simulink model "hardware1"  (R2018a)
settings: Solver=VariableStepAuto  StartTime=0.0  StopTime=10000  RelTol=1e-3
model workspace (MAT data in the model file):
  D = Simulink.Parameter
  D.DataType = 'auto'
  D.Dimensions = [0 0]
libraries: powerlib x15, simulink x1, powerlib_meascontrol x1
settings Model: Creator=yusuf  LastModifiedBy=yusuf

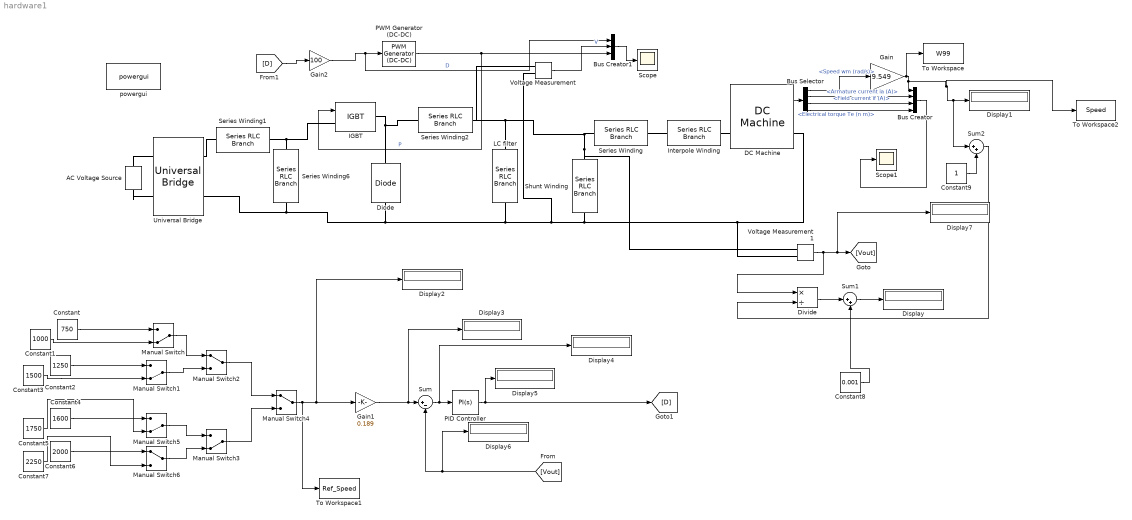
== system hardware1 ==
  AC Voltage Source : powerlib/Electrical Sources/AC Voltage Source  Amplitude=325.27  Phase=0  Frequency=50  SampleTime=0  Measurements=None  BusType=swing  Pref=10e3  Qref=0  Qmin=-inf  Qmax=+inf
  Bus Creator : BusCreator  Inputs=4
  Bus Creator1 : BusCreator  Inputs=3
  Bus Selector : BusSelector  OutputSignals=Speed wm (rad/s),Armature current ia (A),Field current if (A),Electrical torque Te (n m)
  Constant : Constant  Value=750
  Constant1 : Constant  Value=1000
  Constant2 : Constant  Value=1250
  Constant3 : Constant  Value=1500
  Constant4 : Constant  Value=1600
  Constant5 : Constant  Value=1750
  Constant6 : Constant  Value=2000
  Constant7 : Constant  Value=2250
  Constant8 : Constant  Value=0.001
  Constant9 : Constant
  DC Machine : powerlib/Machines/DC Machine  PresetModel=No  MechanicalLoad=Torque TL  FieldType=Permanent magnet  ShowDetailedParameters=on  MeasurementBus=off  RLa=[ 28 0.0133]  RLf="[ 240  120]"  Laf=1.8  MachineConstant=Torque constant (N.m/A)  Ke=1.8  Kt=1.8  J=1  Bm=0  Tf=0  w0=0  Ifinit=1  TsPowergui=0  TsBlock=-1
  Diode : powerlib/Power Electronics/Diode  Ron=0.001  Lon=0  Vf=0.8  IC=0  UseSnubber=0  Rs=500  Cs=250e-9  Measurements=off
  Display{,1..7} (8 alike) : Display
  Divide : Product  Inputs=*/  OutMin=[0.00001]
  Gain : Gain  Gain=9.549
  Gain1 : Gain  Gain=0.189
  Gain2 : Gain  Gain=100
  IGBT : powerlib/Power Electronics/IGBT  Ron=0.001  Lon=0  Vf=1  Tf=1e-6  Tt=2e-6  IC=0  Rs=1e5  Cs=inf  Measurements=off
  Interpole Winding : powerlib/Elements/Series RLC Branch  LConnTagsString=__new0  RConnTagsString=__new0  BranchType=RL  Resistance=0.8  Inductance=0.0058  SetiL0=off  InitialCurrent=0  Capacitance=1e-6  Setx0=off  InitialVoltage=0  Measurements=None
  LC filter : powerlib/Elements/Series RLC Branch  LConnTagsString=__new0  RConnTagsString=__new0  BranchType=C  Resistance=8260  Inductance=6.4  SetiL0=off  InitialCurrent=0  Capacitance=1  Setx0=off  InitialVoltage=0  Measurements=None
  Manual Switch{,1,3,5} (4 alike) : ManualSwitch  CurrentSetting=0
  Manual Switch2 : ManualSwitch
  Manual Switch4 : ManualSwitch
  Manual Switch6 : ManualSwitch
  PID Controller : simulink/Continuous/PID Controller  Controller=PI  TimeDomain=Continuous-time  SampleTime=-1  IntegratorMethod=Forward Euler  FilterMethod=Forward Euler  Form=Parallel  UseFilter=on  ControllerParametersSource=internal  P=5  I=50  D=0  N=100  InitialConditionSource=internal  InitialConditionForIntegrator=0  InitialConditionForFilter=0  ExternalReset=none  LimitOutput=on  UpperSaturationLimit=1  LowerSaturationLimit=0  LinearizeAsGain=on  AntiWindupMode=clamping  Kb=1  TrackingMode=off  Kt=1  PParamMin=[]  PParamMax=[]  IParamMin=[]  IParamMax=[]  DParamMin=[]  DParamMax=[]  NParamMin=[]  NParamMax=[]  KbParamMin=[]  KbParamMax=[]  KtParamMin=[]  KtParamMax=[]  POutMin=[]  POutMax=[]  IOutMin=[]  IOutMax=[]  DOutMin=[]  DOutMax=[]  NOutMin=[]  NOutMax=[]  KbOutMin=[]  KbOutMax=[]  KtOutMin=[]  KtOutMax=[]  IntegratorOutMin=[]  IntegratorOutMax=[]  FilterOutMin=[]  FilterOutMax=[]  SumOutMin=[]  SumOutMax=[]  SumI1OutMin=[]  SumI1OutMax=[]  SumI2OutMin=[]  SumI2OutMax=[]  SumI3OutMin=[]  SumI3OutMax=[]  SumDOutMin=[]  SumDOutMax=[]  SaturationOutMin=[]  SaturationOutMax=[]  IntegratorContinuousStateAttributes=''  IntegratorStateMustResolveToSignalObject=off  IntegratorRTWStateStorageClass=Auto  FilterContinuousStateAttributes=''  FilterStateMustResolveToSignalObject=off  FilterRTWStateStorageClass=Auto  DifferentiatorICPrevScaledInput=0  DifferentiatorOutMin=[]  DifferentiatorOutMax=[]  FilterDiffOutCoefMin=[]  FilterDiffOutCoefMax=[]  SumDenOutMin=[]  SumDenOutMax=[]  SumNumOutMin=[]  SumNumOutMax=[]  ReciprocalOutMin=[]  ReciprocalOutMax=[]  DivideOutMin=[]  DivideOutMax=[]  TunerSelectOption=Transfer Function Based (PID Tuner App)
  PWM Generator (DC-DC) : powerlib_meascontrol/Pulse & Signal Generators/PWM Generator (DC-DC)  Fsw=100  Ts=0
  Scope : Scope
  Scope1 : Scope
  Series Winding : powerlib/Elements/Series RLC Branch  LConnTagsString=__new0  RConnTagsString=__new0  BranchType=RL  Resistance=0.065  Inductance=260e-6  SetiL0=off  InitialCurrent=0  Capacitance=1e-6  Setx0=off  InitialVoltage=0  Measurements=None
  Series Winding1 : powerlib/Elements/Series RLC Branch  LConnTagsString=__new0  RConnTagsString=__new0  BranchType=L  Resistance=0.065  Inductance=100e-3  SetiL0=off  InitialCurrent=0  Capacitance=1e-3  Setx0=off  InitialVoltage=0  Measurements=None
  Series Winding2 : powerlib/Elements/Series RLC Branch  LConnTagsString=__new0  RConnTagsString=__new0  BranchType=RL  Resistance=0.01  Inductance=1  SetiL0=off  InitialCurrent=0  Capacitance=1e-6  Setx0=off  InitialVoltage=0  Measurements=None
  Series Winding6 : powerlib/Elements/Series RLC Branch  LConnTagsString=__new0  RConnTagsString=__new0  BranchType=C  Resistance=0.065  Inductance=260e-6  SetiL0=off  InitialCurrent=0  Capacitance=1.1e-3  Setx0=off  InitialVoltage=0  Measurements=None
  Shunt Winding : powerlib/Elements/Series RLC Branch  LConnTagsString=__new0  RConnTagsString=__new0  BranchType=RL  Resistance=8260  Inductance=6.4  SetiL0=off  InitialCurrent=0  Capacitance=1e-6  Setx0=off  InitialVoltage=0  Measurements=None
  Sum : Sum  Inputs=|+-
  Sum1 : Sum  Inputs=|++
  Sum2 : Sum  Inputs=|++
  To Workspace : ToWorkspace  VariableName=W99  SaveFormat=Timeseries  SampleTime=-1
  To Workspace1 : ToWorkspace  VariableName=Ref_Speed  SaveFormat=Timeseries  SampleTime=-1
  To Workspace2 : ToWorkspace  VariableName=Speed  SaveFormat=Timeseries  SampleTime=-1
  Universal Bridge : powerlib/Power Electronics/Universal Bridge  Arms=2  SnubberResistance=1e5  SnubberCapacitance=inf  Device=Diodes  Ron=1e-3  Lon=0  ForwardVoltages="[  0  0  ]"  ForwardVoltage=0.7  GTOparameters=[ 10e-6 , 20e-6 ]  IGBTparameters=[ 1e-6 , 2e-6 ]  Measurements=None  Measurements_2=None  converterType=Rectifier
  Voltage Measurement : powerlib/Measurements/Voltage Measurement  PhasorSimulation=off  OutputType=Complex  PSBequivalent=0
  Voltage Measurement1 : powerlib/Measurements/Voltage Measurement  PhasorSimulation=off  OutputType=Complex  PSBequivalent=0
  powergui : powerlib/powergui  Priority=1  SimulationMode=Discrete  SampleTime=5e-3  frequency=60  Iterations=50  frequencyindice=0  Pbase=100e6  ErrMax=1e-4  UnitsV=kV  UnitsW=MW  buscounter=0  FunctionMessages=off  echomessages=off  EnableUseOfTLC=off  CurrentSourceSwitches=off  DisableSnubberDevices=off  DisableRonSwitches=off  DisableVfSwitches=off  DisplayEquations=off  SolverType=Tustin/Backward Euler (TBE)  Interpol=off  ExternalGateDelay=off  methode=off  Ts=100  x0status=blocks  SPID=on  SwTol=0  HookPort=off  RestoreLinks=warning  ResistiveCurrentMeasurement=off  Frange=[0:2:500]  Ylog=off  Xlog=on  ShowGrid=off  save=off  variable=ZData  structure=0  ZoomFFT=off  StartTime=0.0  cycles=1  DisplayStyle=1  fundamental=60  FreqAxis=off  MaxFrequency=1000  frequencyindicesteady=1  RmsSteady=1  display=off
  wires:
  DC Machine/1 -> Bus Selector/1
  Bus Creator/1 -> Scope1/1
  Bus Selector/2 -> Bus Creator/2  "<Armature current ia (A)>"
  Bus Selector/3 -> Bus Creator/3  "<Field current if (A)>"
  Bus Selector/4 -> Bus Creator/4  "<Electrical torque Te (n m)>"
  Bus Selector/1 -> Gain/1  "<Speed wm (rad/s)>"
  Gain/1 -> To Workspace/1, To Workspace2/1, Sum2/1, Display1/1, Bus Creator/1
  Voltage Measurement1/1 -> Display7/1, [Vout], Divide/1
  Manual Switch3/1 -> Manual Switch4/2
  Manual Switch2/1 -> Manual Switch4/1
  Manual Switch/1 -> Manual Switch2/1
  Manual Switch1/1 -> Manual Switch2/2
  Manual Switch5/1 -> Manual Switch3/1
  Manual Switch6/1 -> Manual Switch3/2
  Constant/1 -> Manual Switch/1
  Constant1/1 -> Manual Switch/2
  Constant2/1 -> Manual Switch1/1
  Constant3/1 -> Manual Switch1/2
  Constant4/1 -> Manual Switch5/1
  Constant5/1 -> Manual Switch5/2
  Constant6/1 -> Manual Switch6/1
  Constant7/1 -> Manual Switch6/2
  Manual Switch4/1 -> To Workspace1/1, Gain1/1, Display2/1
  Sum/1 -> Display4/1, PID Controller/1
  Gain1/1 -> Display3/1, Sum/1
  [Vout] -> Display6/1, Sum/2
  PWM Generator (DC-DC)/1 -> Bus Creator1/3, IGBT/1  "P"
  [D] -> Gain2/1
  Gain2/1 -> Bus Creator1/1, PWM Generator (DC-DC)/1  "D"
  PID Controller/1 -> [D], Display5/1
  Constant9/1 -> Sum2/2
  Sum2/1 -> Divide/2
  Divide/1 -> Sum1/1
  Sum1/1 -> Display/1
  Constant8/1 -> Sum1/2
  Voltage Measurement/1 -> Bus Creator1/2  "V"
  Bus Creator1/1 -> Scope/1
  connections:
  Interpole Winding/RConn1 -- DC Machine/LConn1
  Series Winding/RConn1 -- Interpole Winding/LConn1
  AC Voltage Source/RConn1 -- Universal Bridge/LConn1
  AC Voltage Source/LConn1 -- Universal Bridge/LConn2
  DC Machine/RConn1 -- Voltage Measurement1/LConn2 -- Voltage Measurement/LConn2 -- LC filter/LConn1 -- Series Winding6/RConn1 -- Universal Bridge/RConn2 -- Diode/LConn1 -- Shunt Winding/LConn1
  Series Winding1/RConn1 -- Universal Bridge/RConn1
  IGBT/RConn1 -- Series Winding2/LConn1 -- Diode/RConn1
  Series Winding1/LConn1 -- IGBT/LConn1 -- Series Winding6/LConn1
  Series Winding2/RConn1 -- Voltage Measurement1/LConn1 -- Shunt Winding/RConn1 -- Series Winding/LConn1 -- Voltage Measurement/LConn1 -- LC filter/RConn1
